simulink model "Segunda_lei_de_controle"  (R2015b)
settings: Solver=VariableStepAuto  StartTime=0.0  StopTime=10.0  RelTol=1e-3
settings Model: Creator=egidio.neto  LastModifiedBy=egidio.neto

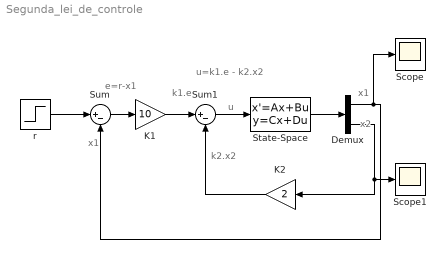
== system Segunda_lei_de_controle ==
  note: u
  note: k1.e
  note: k2.x2
  note: e=r-x1
  note: x1
  note: x2
  note: x1
  note: u=k1.e - k2.x2
  Demux : Demux  Outputs=2
  K1 : Gain  Gain=10
  K2 : Gain  Gain=2
  Scope : Scope
  Scope1 : Scope
  State-Space : StateSpace  A=[0 1; 0 -2]  B=[0;1]  C=[1 0; 0 1]  D=[0;0]  X0=[0; 0]
  Sum : Sum  Inputs=|+-
  Sum1 : Sum  Inputs=|+-
  r : Step  SampleTime=0
  wires:
  State-Space/1 -> Demux/1
  r/1 -> Sum/1
  Demux/1 -> Scope/1, Sum/2
  Sum/1 -> K1/1
  K1/1 -> Sum1/1
  Demux/2 -> Scope1/1, K2/1
  K2/1 -> Sum1/2
  Sum1/1 -> State-Space/1
